simulink model "teste"  (R2012b)
settings: Solver=ode45  StartTime=0.0  StopTime=1  RelTol=1e-3
libraries: Tools x6, simulink x6, BLDC x4
settings Model: Creator=h3now  LastModifiedBy=h3now

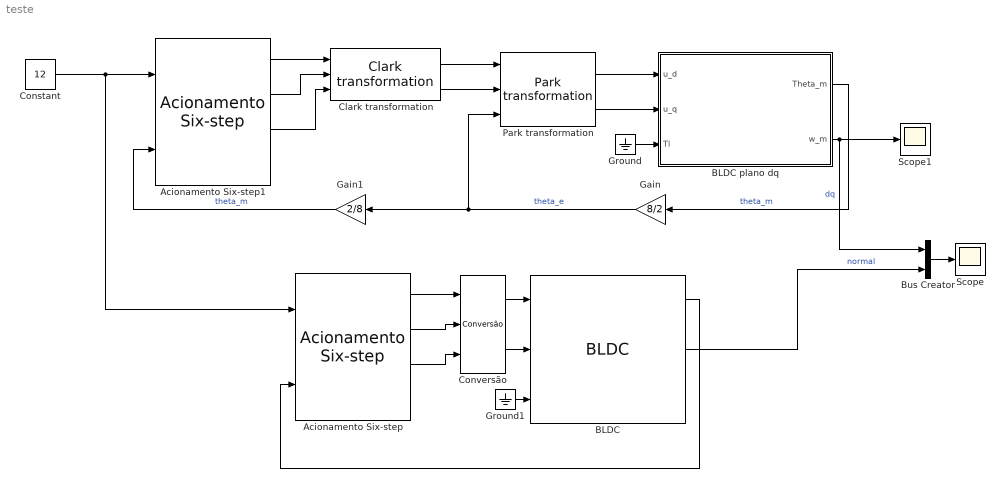
== system teste ==
  Acionamento Six-step : BLDC/Acionamento Six-step  P=8
  Acionamento Six-step1 : BLDC/Acionamento Six-step  P=8
  BLDC : BLDC/BLDC  J=1.39e-6  R=10.1/2  L=2.04/2000  P=8  Kt=15.7e-3/1.19  Ke=15.7e-3/1.19  Kd=0  default_fcem=on  fcem_a=fcem_a  fcem_b=fcem_b  fcem_c=fcem_c
  BLDC plano dq : Subsystem  mask{J=1.39e-6, R=10.1/2, L=2.04/2000, P=8, Kt=15.7e-3/1.19, Ke=15.7e-3/1.19, Kd=0, default_fcem=on, fcem_a=0, fcem_b=0, fcem_c=0}
      mask prompts: J "Inércia do sistema motor+carga"; R "Resistência por Fase"; L "Indutância por fase"; P "Número de pólos"; Kt "Constante de torque"; Ke "Constante de força eletromotriz"; Kd "Constante de atrito viscoso"; default_fcem "Utilizar back-emf padrão?"; fcem_a "Forma da back-emf na fase a"; fcem_b "Forma da back-emf na fase b"; fcem_c "Forma da back-emf na fase c"
      mask init:
      | % Se o usuário escolheu utilizar a back-emf padrão, inicializa as variáveis
      | % da lookuptables com valores zerados para não dar erro.
      | if default_fcem == 1
      |     fcem_a = [0,0;1,0];
      |     fcem_b = [0,0;1,0];
      |     fcem_c = [0,0;1,0];
      |     
      | % Se o usuário escolheu especificar qual será a forma da back-emf, checa se
      | % as lookup tables que ele inseriu fazem sentido.
      | else
      |     % Checa se a primeira coluna começa em 0.
      |     if fcem_a(1,1) ~= 0 ||fcem_b(1,1) ~= 0 || fcem_c(1,1) ~= 0
      |         error('A primeira coluna das lookup tables que definem o formato da back-emf devem começar em zero!');
      |     end
      |     % Checa se a primeira coluna termina em 360.
      |     if fcem_a(size(fcem_a,1),1) ~= 360 || fcem_b(size(fcem_b,1),1) ~= 360 || fcem_c(size(fcem_c,1),1) ~= 360
      |         error('A primeira coluna das lookup tables que definem o formato da back-emf deve terminar em 360!');
      |     end
      | end
      mask Callback default_fcem:
      | maskStr = get_param(gcb,'MaskValues');
      | 
      | if strcmp(maskStr{8},'on')
      |     set_param(gcb,'MaskVisibilities',{'on';'on';'on';'on';'on';'on';'on';'on';'off';'off';'off'});
      | else
      |     set_param(gcb,'MaskVisibilities',{'on';'on';'on';'on';'on';'on';'on';'on';'on';'on';'on'});
      | end
  Bus Creator : BusCreator  Inputs=2
  Clark transformation : Tools/Clark transformation
  Constant : Constant  Value=12
  Conversão : BLDC/Conversão
  Gain : Gain  Gain=8/2
  Gain1 : Gain  Gain=2/8
  Ground : Ground
  Ground1 : Ground
  Park transformation : Tools/Park transformation
  Scope : Scope
      settings: ShowLegends=on
  Scope1 : Scope
      settings: ShowLegends=on  YMin=875  YMax=1150
  wires:
  Clark transformation/1 -> Park transformation/1
  Clark transformation/2 -> Park transformation/2
  Acionamento Six-step1/1 -> Clark transformation/1
  Acionamento Six-step1/2 -> Clark transformation/2
  Acionamento Six-step1/3 -> Clark transformation/3
  BLDC/1 -> Acionamento Six-step/2
  Ground/1 -> BLDC plano dq/3(Tl)
  Ground1/1 -> BLDC/3
  Constant/1 -> Acionamento Six-step/1, Acionamento Six-step1/1
  Bus Creator/1 -> Scope/1
  BLDC plano dq/2(w_m) -> Bus Creator/1, Scope1/1  "dq"
  BLDC/2 -> Bus Creator/2  "normal"
  BLDC plano dq/1(Theta_m) -> Gain/1  "theta_m"
  Gain/1 -> Gain1/1, Park transformation/3  "theta_e"
  Gain1/1 -> Acionamento Six-step1/2  "theta_m"
  Park transformation/1 -> BLDC plano dq/1(u_d)
  Park transformation/2 -> BLDC plano dq/2(u_q)
  Conversão/1 -> BLDC/1
  Conversão/2 -> BLDC/2
  Acionamento Six-step/1 -> Conversão/1
  Acionamento Six-step/2 -> Conversão/2
  Acionamento Six-step/3 -> Conversão/3

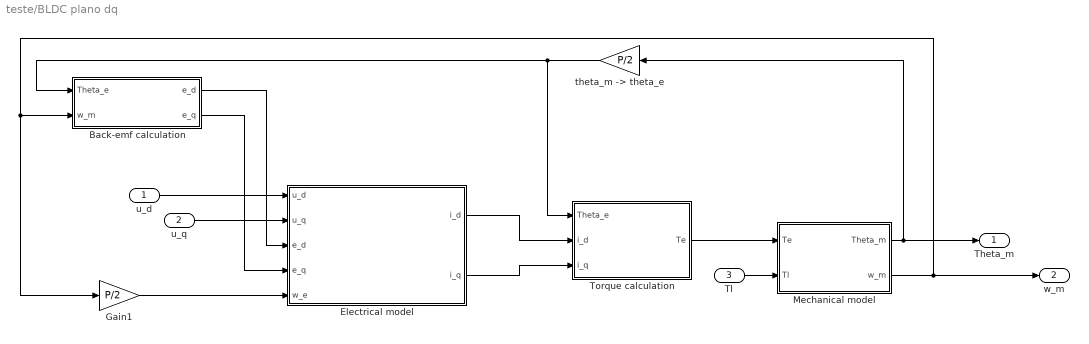
== system teste/BLDC plano dq ==
  u_d : Inport
  u_q : Inport  Port=2
  Tl : Inport  Port=3
  Back-emf calculation : Subsystem
  Electrical model : Subsystem
  Gain1 : Gain  Gain=P/2
  Mechanical model : Subsystem
  Torque calculation : Subsystem
  "theta_m -> theta_e" : Gain  Gain=P/2
  Theta_m : Outport
  w_m : Outport  Port=2
  wires:
  Back-emf calculation/2(e_q) -> Electrical model/4(e_q)
  u_q/1 -> Electrical model/2(u_q)
  Tl/1 -> Mechanical model/2(Tl)
  Mechanical model/2(w_m) -> w_m/1, Back-emf calculation/2(w_m), Gain1/1
  Mechanical model/1(Theta_m) -> Theta_m/1, "theta_m -> theta_e"/1
  "theta_m -> theta_e"/1 -> Torque calculation/1(Theta_e), Back-emf calculation/1(Theta_e)
  Gain1/1 -> Electrical model/5(w_e)
  u_d/1 -> Electrical model/1(u_d)
  Back-emf calculation/1(e_d) -> Electrical model/3(e_d)
  Electrical model/1(i_d) -> Torque calculation/2(i_d)
  Electrical model/2(i_q) -> Torque calculation/3(i_q)
  Torque calculation/1(Te) -> Mechanical model/1(Te)

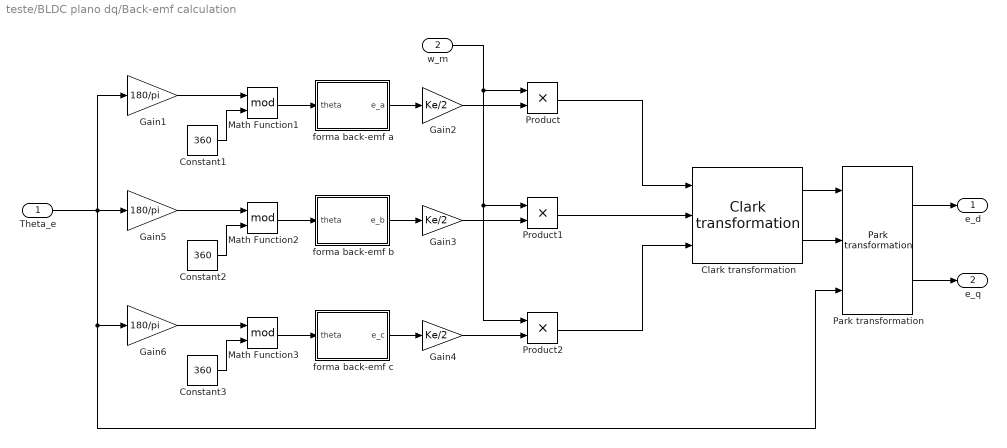
== system teste/BLDC plano dq/Back-emf calculation ==
  Theta_e : Inport
  w_m : Inport  Port=2
  Clark transformation : Tools/Clark transformation
  Constant1 : Constant  Value=360
  Constant2 : Constant  Value=360
  Constant3 : Constant  Value=360
  Gain1 : Gain  Gain=180/pi
  Gain2 : Gain  Gain=Ke/2
  Gain3 : Gain  Gain=Ke/2
  Gain4 : Gain  Gain=Ke/2
  Gain5 : Gain  Gain=180/pi
  Gain6 : Gain  Gain=180/pi
  Math Function1 : Math  Operator=mod  SaturateOnIntegerOverflow=on
  Math Function2 : Math  Operator=mod  SaturateOnIntegerOverflow=on
  Math Function3 : Math  Operator=mod  SaturateOnIntegerOverflow=on
  Park transformation : Tools/Park transformation
  Product : Product  RndMeth=Zero
  Product1 : Product  RndMeth=Zero
  Product2 : Product  RndMeth=Zero
  forma back-emf a : Subsystem
  forma back-emf b : Subsystem
  forma back-emf c : Subsystem
  e_d : Outport
  e_q : Outport  Port=2
  wires:
  forma back-emf c/1(e_c) -> Gain4/1
  Math Function3/1 -> forma back-emf c/1(theta)
  forma back-emf b/1(e_b) -> Gain3/1
  Math Function2/1 -> forma back-emf b/1(theta)
  forma back-emf a/1(e_a) -> Gain2/1
  Math Function1/1 -> forma back-emf a/1(theta)
  Gain6/1 -> Math Function3/1
  Gain5/1 -> Math Function2/1
  Gain1/1 -> Math Function1/1
  Gain4/1 -> Product2/2
  Gain3/1 -> Product1/2
  w_m/1 -> Product2/1, Product1/1, Product/1
  Gain2/1 -> Product/2
  Product2/1 -> Clark transformation/3
  Product1/1 -> Clark transformation/2
  Product/1 -> Clark transformation/1
  Constant1/1 -> Math Function1/2
  Constant2/1 -> Math Function2/2
  Constant3/1 -> Math Function3/2
  Clark transformation/1 -> Park transformation/1
  Clark transformation/2 -> Park transformation/2
  Park transformation/1 -> e_d/1
  Park transformation/2 -> e_q/1
  Theta_e/1 -> Gain6/1, Park transformation/3, Gain1/1, Gain5/1

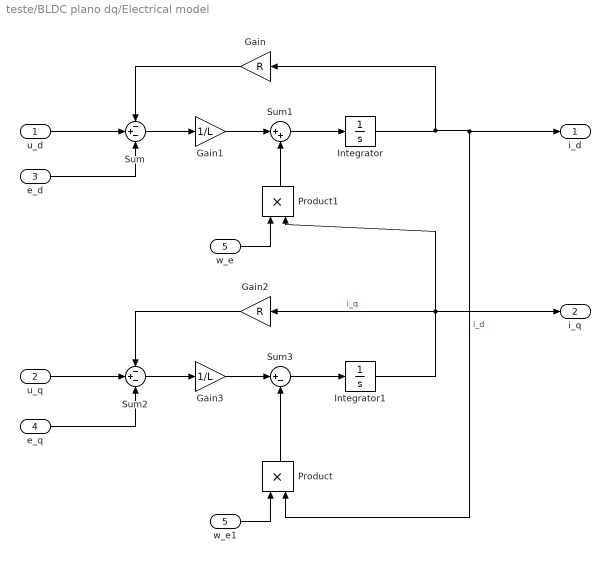
== system teste/BLDC plano dq/Electrical model ==
  u_d : Inport
  u_q : Inport  Port=2
  e_d : Inport  Port=3
  e_q : Inport  Port=4
  w_e : Inport  Port=5
  Gain : Gain  Gain=R
  Gain1 : Gain  Gain=1/L
  Gain2 : Gain  Gain=R
  Gain3 : Gain  Gain=1/L
  Integrator : Integrator
  Integrator1 : Integrator
  Product : Product  RndMeth=Zero
  Product1 : Product  RndMeth=Zero
  Sum : Sum  Inputs=-+-
  Sum1 : Sum  Inputs=|++
  Sum2 : Sum  Inputs=-+-
  Sum3 : Sum  Inputs=|+-
  w_e1 : InportShadow  Port=5
  i_d : Outport
  i_q : Outport  Port=2
  wires:
  Product/1 -> Sum3/2
  Sum3/1 -> Integrator1/1
  Gain3/1 -> Sum3/1
  Integrator1/1 -> i_q/1, Gain2/1, Product1/2  "i_q"
  Gain2/1 -> Sum2/1
  u_q/1 -> Sum2/2
  e_q/1 -> Sum2/3
  Sum2/1 -> Gain3/1
  Product1/1 -> Sum1/2
  Sum1/1 -> Integrator/1
  Integrator/1 -> i_d/1, Product/2, Gain/1  "i_d"
  e_d/1 -> Sum/3
  Gain/1 -> Sum/1
  Sum/1 -> Gain1/1
  Gain1/1 -> Sum1/1
  u_d/1 -> Sum/2
  w_e/1 -> Product1/1
  w_e1/1 -> Product/1

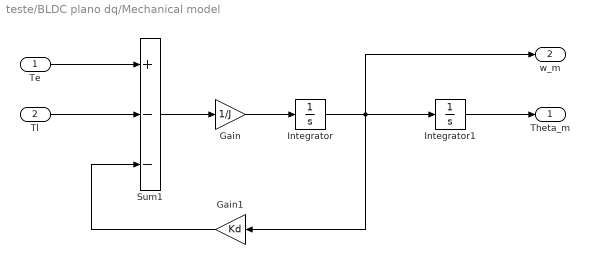
== system teste/BLDC plano dq/Mechanical model ==
  Te : Inport
  Tl : Inport  Port=2
  Gain : Gain  Gain=1/J
  Gain1 : Gain  Gain=Kd
  Integrator : Integrator
  Integrator1 : Integrator
  Sum1 : Sum  Inputs=+--
  Theta_m : Outport
  w_m : Outport  Port=2
  wires:
  Sum1/1 -> Gain/1
  Gain/1 -> Integrator/1
  Integrator/1 -> w_m/1, Integrator1/1, Gain1/1
  Te/1 -> Sum1/1
  Gain1/1 -> Sum1/3
  Tl/1 -> Sum1/2
  Integrator1/1 -> Theta_m/1

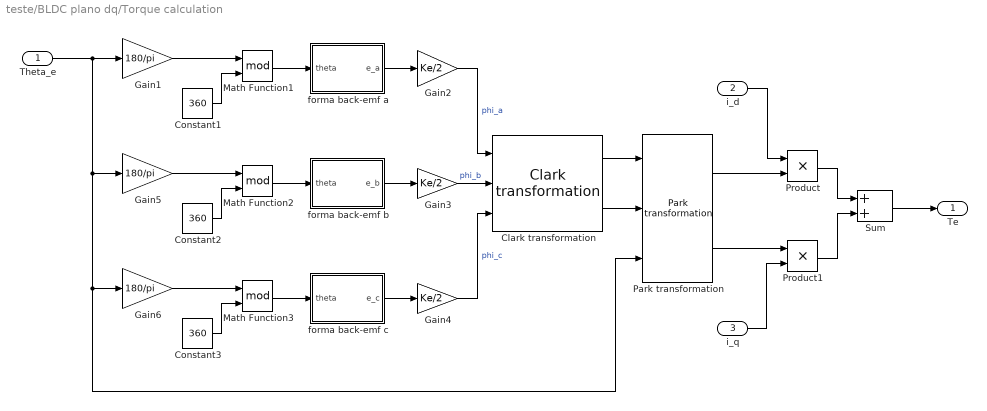
== system teste/BLDC plano dq/Torque calculation ==
  Theta_e : Inport
  i_d : Inport  Port=2
  i_q : Inport  Port=3
  Clark transformation : Tools/Clark transformation
  Constant1 : Constant  Value=360
  Constant2 : Constant  Value=360
  Constant3 : Constant  Value=360
  Gain1 : Gain  Gain=180/pi
  Gain2 : Gain  Gain=Ke/2
  Gain3 : Gain  Gain=Ke/2
  Gain4 : Gain  Gain=Ke/2
  Gain5 : Gain  Gain=180/pi
  Gain6 : Gain  Gain=180/pi
  Math Function1 : Math  Operator=mod  SaturateOnIntegerOverflow=on
  Math Function2 : Math  Operator=mod  SaturateOnIntegerOverflow=on
  Math Function3 : Math  Operator=mod  SaturateOnIntegerOverflow=on
  Park transformation : Tools/Park transformation
  Product : Product  RndMeth=Zero
  Product1 : Product  RndMeth=Zero
  Sum : Sum
  forma back-emf a : Subsystem
  forma back-emf b : Subsystem
  forma back-emf c : Subsystem
  Te : Outport
  wires:
  forma back-emf c/1(e_c) -> Gain4/1
  Math Function3/1 -> forma back-emf c/1(theta)
  forma back-emf b/1(e_b) -> Gain3/1
  Math Function2/1 -> forma back-emf b/1(theta)
  forma back-emf a/1(e_a) -> Gain2/1
  Math Function1/1 -> forma back-emf a/1(theta)
  Gain6/1 -> Math Function3/1
  Gain5/1 -> Math Function2/1
  Gain1/1 -> Math Function1/1
  Gain4/1 -> Clark transformation/3  "phi_c"
  Gain3/1 -> Clark transformation/2  "phi_b"
  Gain2/1 -> Clark transformation/1  "phi_a"
  Constant1/1 -> Math Function1/2
  Constant2/1 -> Math Function2/2
  Constant3/1 -> Math Function3/2
  Clark transformation/1 -> Park transformation/1
  Clark transformation/2 -> Park transformation/2
  Theta_e/1 -> Gain6/1, Park transformation/3, Gain5/1, Gain1/1
  Park transformation/1 -> Product/2
  i_d/1 -> Product/1
  i_q/1 -> Product1/2
  Park transformation/2 -> Product1/1
  Product/1 -> Sum/1
  Product1/1 -> Sum/2
  Sum/1 -> Te/1

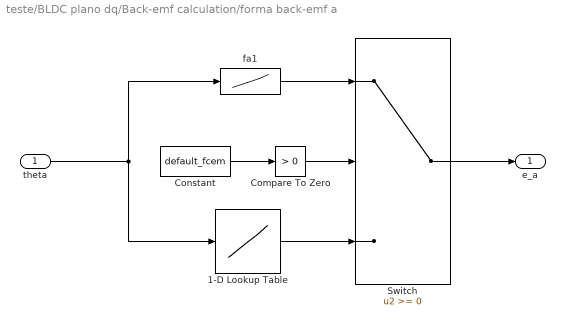
== system teste/BLDC plano dq/Back-emf calculation/forma back-emf a ==
  theta : Inport
  1-D Lookup Table : Lookup_n-D  NumberOfTableDimensions=1  BreakpointsForDimension1=fcem_a(:,1)  Table=fcem_a(:,2)  RndMeth=Simplest  InputSameDT=on
  Compare To Zero : simulink/Logic and Bit Operations/Compare To Zero  relop=>  OutDataTypeStr=boolean
  Constant : Constant  Value=default_fcem
  Switch : Switch
  fa1 : Lookup  InputValues=[0 30 60 90 120 150 180 210 240 270 300 330 360]  Table=[ 1 1 1 0 -1 -1 -1 -1 -1 0 1 1 1]
  e_a : Outport
  wires:
  Constant/1 -> Compare To Zero/1
  Compare To Zero/1 -> Switch/2
  1-D Lookup Table/1 -> Switch/3
  fa1/1 -> Switch/1
  Switch/1 -> e_a/1
  theta/1 -> fa1/1, 1-D Lookup Table/1

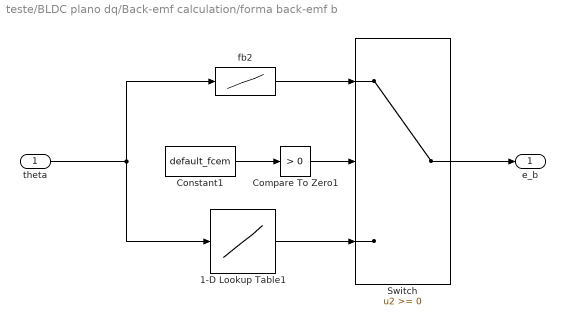
== system teste/BLDC plano dq/Back-emf calculation/forma back-emf b ==
  theta : Inport
  1-D Lookup Table1 : Lookup_n-D  NumberOfTableDimensions=1  BreakpointsForDimension1=fcem_b(:,1)  Table=fcem_b(:,2)  RndMeth=Simplest  InputSameDT=on
  Compare To Zero1 : simulink/Logic and Bit Operations/Compare To Zero  relop=>  OutDataTypeStr=boolean
  Constant1 : Constant  Value=default_fcem
  Switch : Switch
  fb2 : Lookup  InputValues=[0 30 60 90 120 150 180 210 240 270 300 330 360]  Table=[-1 0 1 1 1 1 1 0 -1 -1 -1 -1 -1]
  e_b : Outport
  wires:
  fb2/1 -> Switch/1
  Switch/1 -> e_b/1
  Constant1/1 -> Compare To Zero1/1
  Compare To Zero1/1 -> Switch/2
  theta/1 -> fb2/1, 1-D Lookup Table1/1
  1-D Lookup Table1/1 -> Switch/3

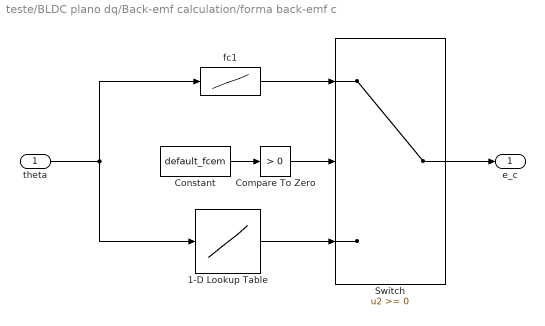
== system teste/BLDC plano dq/Back-emf calculation/forma back-emf c ==
  theta : Inport
  1-D Lookup Table : Lookup_n-D  NumberOfTableDimensions=1  BreakpointsForDimension1=fcem_c(:,1)  Table=fcem_c(:,2)  RndMeth=Simplest  InputSameDT=on
  Compare To Zero : simulink/Logic and Bit Operations/Compare To Zero  relop=>  OutDataTypeStr=boolean
  Constant : Constant  Value=default_fcem
  Switch : Switch
  fc1 : Lookup  InputValues=[0 30 60 90 120 150 180 210 240 270 300 330 360]  Table=[-1 -1 -1 -1 -1 0 1 1 1 1 1 0 -1]
  e_c : Outport
  wires:
  fc1/1 -> Switch/1
  Switch/1 -> e_c/1
  Constant/1 -> Compare To Zero/1
  Compare To Zero/1 -> Switch/2
  theta/1 -> fc1/1, 1-D Lookup Table/1
  1-D Lookup Table/1 -> Switch/3

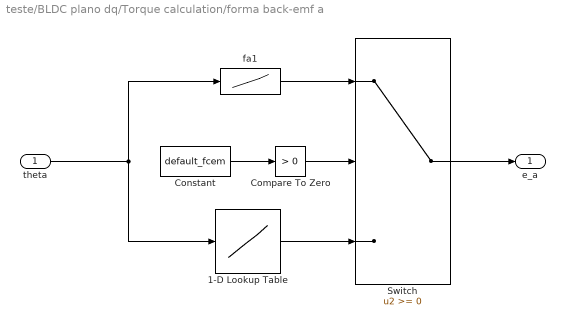
== system teste/BLDC plano dq/Torque calculation/forma back-emf a ==
  theta : Inport
  1-D Lookup Table : Lookup_n-D  NumberOfTableDimensions=1  BreakpointsForDimension1=fcem_a(:,1)  Table=fcem_a(:,2)  RndMeth=Simplest  InputSameDT=on
  Compare To Zero : simulink/Logic and Bit Operations/Compare To Zero  relop=>  OutDataTypeStr=boolean
  Constant : Constant  Value=default_fcem
  Switch : Switch
  fa1 : Lookup  InputValues=[0 30 60 90 120 150 180 210 240 270 300 330 360]  Table=[ 1 1 1 0 -1 -1 -1 -1 -1 0 1 1 1]
  e_a : Outport
  wires:
  Constant/1 -> Compare To Zero/1
  Compare To Zero/1 -> Switch/2
  1-D Lookup Table/1 -> Switch/3
  fa1/1 -> Switch/1
  Switch/1 -> e_a/1
  theta/1 -> fa1/1, 1-D Lookup Table/1

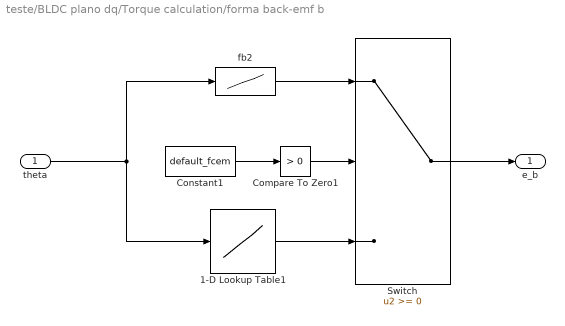
== system teste/BLDC plano dq/Torque calculation/forma back-emf b ==
  theta : Inport
  1-D Lookup Table1 : Lookup_n-D  NumberOfTableDimensions=1  BreakpointsForDimension1=fcem_b(:,1)  Table=fcem_b(:,2)  RndMeth=Simplest  InputSameDT=on
  Compare To Zero1 : simulink/Logic and Bit Operations/Compare To Zero  relop=>  OutDataTypeStr=boolean
  Constant1 : Constant  Value=default_fcem
  Switch : Switch
  fb2 : Lookup  InputValues=[0 30 60 90 120 150 180 210 240 270 300 330 360]  Table=[-1 0 1 1 1 1 1 0 -1 -1 -1 -1 -1]
  e_b : Outport
  wires:
  fb2/1 -> Switch/1
  Switch/1 -> e_b/1
  Constant1/1 -> Compare To Zero1/1
  Compare To Zero1/1 -> Switch/2
  theta/1 -> fb2/1, 1-D Lookup Table1/1
  1-D Lookup Table1/1 -> Switch/3

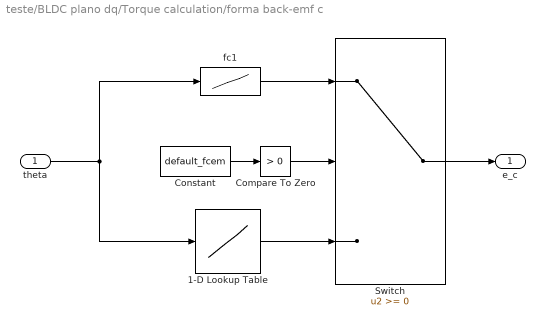
== system teste/BLDC plano dq/Torque calculation/forma back-emf c ==
  theta : Inport
  1-D Lookup Table : Lookup_n-D  NumberOfTableDimensions=1  BreakpointsForDimension1=fcem_c(:,1)  Table=fcem_c(:,2)  RndMeth=Simplest  InputSameDT=on
  Compare To Zero : simulink/Logic and Bit Operations/Compare To Zero  relop=>  OutDataTypeStr=boolean
  Constant : Constant  Value=default_fcem
  Switch : Switch
  fc1 : Lookup  InputValues=[0 30 60 90 120 150 180 210 240 270 300 330 360]  Table=[-1 -1 -1 -1 -1 0 1 1 1 1 1 0 -1]
  e_c : Outport
  wires:
  fc1/1 -> Switch/1
  Switch/1 -> e_c/1
  Constant/1 -> Compare To Zero/1
  Compare To Zero/1 -> Switch/2
  theta/1 -> fc1/1, 1-D Lookup Table/1
  1-D Lookup Table/1 -> Switch/3
